simulink subsystem "cvrs_ventricle"  (R2020b)
settings: Solver=VariableStepAuto  StartTime=0.0  StopTime=10.0  RelTol=1e-3
settings Model: Creator=RH  LastModifiedBy=Marco

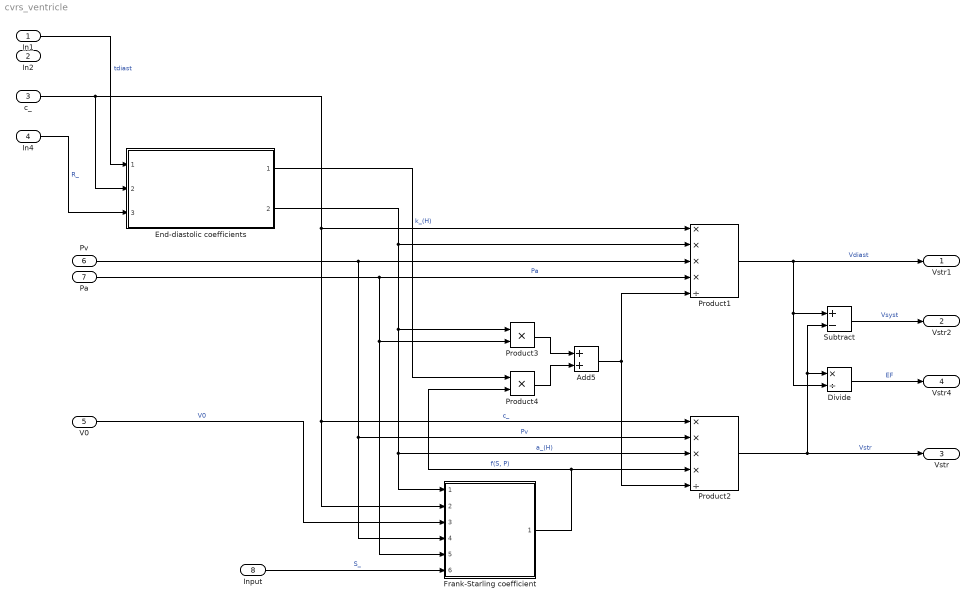
== system cvrs_ventricle ==
  In1 : Inport  Unit=s
  In2 : Inport  Port=2  Unit=s
  c_ : Inport  Port=3  Unit=liter/mmHg
  In4 : Inport  Port=4  Unit=mmHg*min/L
  V0 : Inport  Port=5  Unit=liter
  Pv : Inport  Port=6  Unit=mmHg
  Pa : Inport  Port=7  Unit=mmHg
  Input : Inport  Port=8  Unit=mmHg
  Add5 : Sum
  Divide : Product  Inputs=*/
  End-diastolic coefficients : Subsystem  ReferencedSubsystem=cvrs_diastole_coefficients
  Frank-Starling coefficient : Subsystem  ReferencedSubsystem=cvrs_frank_starling
  Product1 : Product  Inputs=****/
  Product2 : Product  Inputs=****/
  Product3 : Product
  Product4 : Product
  Subtract : Sum  Inputs=+-
  Vstr1 : Outport  Unit=liter
  Vstr2 : Outport  Port=2  Unit=liter
  Vstr : Outport  Port=3  Unit=liter
  Vstr4 : Outport  Port=4  Unit=1
  wires:
  Divide/1 -> Vstr4/1  "EF"
  End-diastolic coefficients/1 -> Product4/1  "k_(H)"
  Product3/1 -> Add5/1
  Pa/1 -> Frank-Starling coefficient/5, Product3/2, Product1/4  "Pa"
  c_/1 -> Product1/1, Frank-Starling coefficient/2, Product2/1, End-diastolic coefficients/2  "c_"
  Frank-Starling coefficient/1 -> Product2/4, Product4/2  "f(S, P)"
  Product4/1 -> Add5/2
  End-diastolic coefficients/2 -> Product1/2, Product3/1, Frank-Starling coefficient/1, Product2/3  "a_(H)"
  Pv/1 -> Frank-Starling coefficient/4, Product2/2, Product1/3  "Pv"
  Add5/1 -> Product2/5, Product1/5
  Product2/1 -> Vstr/1, Subtract/2, Divide/1  "Vstr"
  V0/1 -> Frank-Starling coefficient/3  "V0"
  Product1/1 -> Vstr1/1, Subtract/1, Divide/2  "Vdiast"
  In1/1 -> End-diastolic coefficients/1  "tdiast"
  In4/1 -> End-diastolic coefficients/3  "R_"
  Subtract/1 -> Vstr2/1  "Vsyst"
  Input/1 -> Frank-Starling coefficient/6  "S_"
